simulink model "Quadrotor_Model"  (R2025b)
settings: Solver=ode45  StartTime=0.0  StopTime=15000  RelTol=1e-3  EnableMultiTasking=on
values from neighbouring files (symbols this model uses):
  b = 0.07    [project_launch.m]
  g = 9.81    [project_launch.m]
  Ixx = (2/5) * m_drone * r_body^2 + 2 * L^2 * m_motor    (= 0.0145321875)    [project_launch.m]
  Iyy = Ixx    (= 0.0145321875)    [project_launch.m]
  Izz = (2/5) * m_drone * r_body^2 + 4 * L^2 * m_motor    (= 0.0270321875)    [project_launch.m]
  Jr = 0.01 * m_motor * r_prop^2    (= 1.6129e-05)    [project_launch.m]
  k = 0.09    [project_launch.m]
  K_d_phi = 8    [project_launch.m]
  K_d_psi = 4    [project_launch.m]
  K_d_theta = 8    [project_launch.m]
  K_dx = 1.2    [project_launch.m]
  K_dy = 1.2    [project_launch.m]
  K_dz = 1.8    [project_launch.m]
  K_p_phi = 25    [project_launch.m]
  K_p_psi = 9    [project_launch.m]
  K_p_theta = 25    [project_launch.m]
  K_px = 0.6    [project_launch.m]
  K_py = 0.6    [project_launch.m]
  K_pz = 1.2    [project_launch.m]
  L = 0.25    [project_launch.m]
  m = 1.7006    [project_launch.m]
  tau_v = 0.1    [project_launch.m]
settings Model: Creator=boyan  LastModifiedBy=89286
settings SolverCC: MaxConsecutiveMinStep=2  AlgebraicLoopSolver=TrustRegion
settings DataIOCC: LimitDataPoints=on  SaveFormat=Array  ReturnWorkspaceOutputs=off
settings OptimizationCC: LifeSpan=inf
settings DebuggingCC: SolverPrmCheckMsg=warning  UnconnectedInputMsg=warning  UnconnectedOutputMsg=warning  UnconnectedLineMsg=warning  SFUnexpectedBacktrackingDiag=warning  SFNoUnconditionalDefaultTransitionDiag=warning  SFExecutionAtInitializationDiag=none  ArithmeticOperatorsInVariantConditions=warning
settings HardwareCC: ProdBitPerPointer=32.0  ProdBitPerSizeT=32.0  ProdBitPerPtrDiffT=32.0  ProdLargestAtomicFloat=None  ProdIntDivRoundTo=Undefined  ProdEndianess=Unspecified  ProdWordSize=32.0  ProdHWDeviceType=32-bit Generic
settings ModelReferenceCC: EnableRefExpFcnMdlSchedulingChecks=on  PropagateSignalLabelsOutOfModel=off
settings SFSimCC: SimUseLocalCustomCode=off  CustomCodeUndefinedFunction=UseInterfaceOnly
settings RTWCC: RTWUseLocalCustomCode=off  GPUComputeCapability=3.5  DLArmComputeVersion=19.05
settings CodeAppCC: StateflowObjectComments=on
settings GRTTargetCC: TargetLangStandard=C89/C90 (ANSI)
settings ConfigComp: CovMetricSettings=dw  CovSaveCumulativeToWorkspaceVar=on  CovSaveSingleToWorkspaceVar=on  CovExternalEMLEnable=off  CovSFcnEnable=off

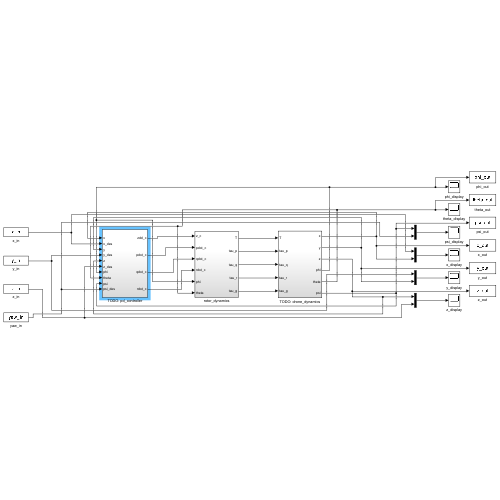
[thumbnail: Simulink's stored preview of the top-level diagram]
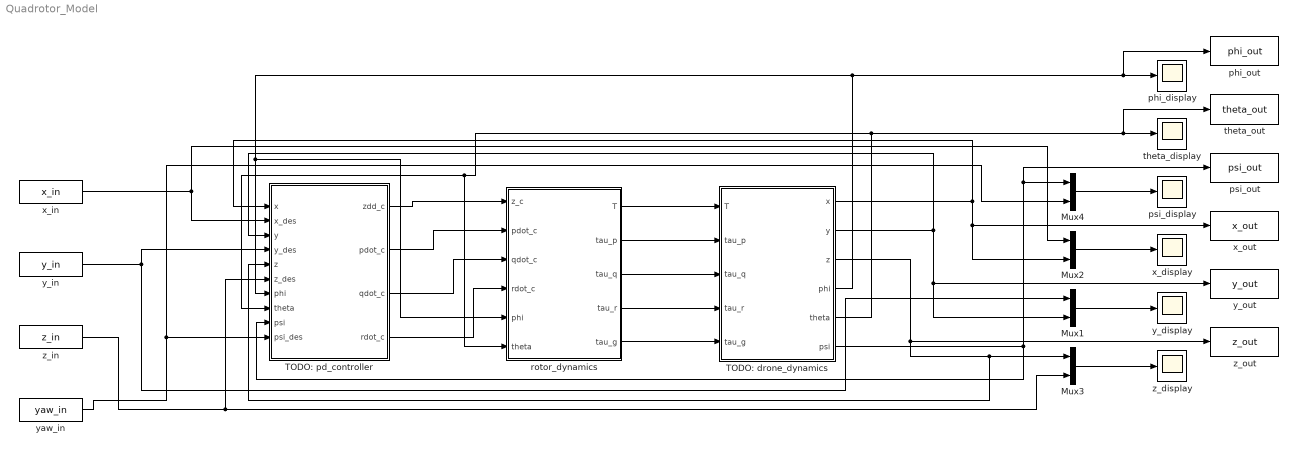
== system Quadrotor_Model ==
  Mux{1..4} (4 alike) : Mux  Inputs=2
  TODO: drone_dynamics : Subsystem
  TODO: pd_controller : Subsystem
  phi_display : Scope
      settings: ActiveDisplayYMinimum=-48.30659  ActiveDisplayYMaximum=31.01137
  phi_out : ToWorkspace  VariableName=phi_out  SaveFormat=Timeseries  SampleTime=-1
  psi_display : Scope
      settings: ActiveDisplayYMinimum=-104019.46579  ActiveDisplayYMaximum=26220.25866  DataLoggingVariableName=ScopeData2
  psi_out : ToWorkspace  VariableName=psi_out  SaveFormat=Timeseries  SampleTime=-1
  rotor_dynamics : Subsystem
  theta_display : Scope
      settings: ActiveDisplayYMinimum=-1.26378  ActiveDisplayYMaximum=0.84614  DataLoggingVariableName=ScopeData3
  theta_out : ToWorkspace  VariableName=theta_out  SaveFormat=Timeseries  SampleTime=-1
  x_display : Scope
      settings: ActiveDisplayYMinimum=-0.02581  ActiveDisplayYMaximum=0.17972  DataLoggingVariableName=ScopeData4
  x_in : FromWorkspace  VariableName=x_in
  x_out : ToWorkspace  VariableName=x_out  SaveFormat=Timeseries  SampleTime=-1
  y_display : Scope
      settings: ActiveDisplayYMinimum=98.09651  ActiveDisplayYMaximum=101.74643  DataLoggingVariableName=ScopeData5
  y_in : FromWorkspace  VariableName=y_in
  y_out : ToWorkspace  VariableName=y_out  SaveFormat=Timeseries  SampleTime=-1
  yaw_in : FromWorkspace  VariableName=yaw_in
  z_display : Scope
      settings: ActiveDisplayYMinimum=-47.57242  ActiveDisplayYMaximum=5.28582
  z_in : FromWorkspace  VariableName=z_in
  z_out : ToWorkspace  VariableName=z_out  SaveFormat=Timeseries  SampleTime=-1
  wires:
  rotor_dynamics/1(T) -> TODO: drone_dynamics/1(T)
  rotor_dynamics/2(tau_p) -> TODO: drone_dynamics/2(tau_p)
  TODO: pd_controller/1(zdd_c) -> rotor_dynamics/1(z_c)
  TODO: pd_controller/2(pdot_c) -> rotor_dynamics/2(pdot_c)
  z_in/1 -> TODO: pd_controller/6(z_des), Mux3/2
  Mux1/1 -> y_display/1
  Mux2/1 -> x_display/1
  Mux4/1 -> psi_display/1
  Mux3/1 -> z_display/1
  TODO: drone_dynamics/6(psi) -> TODO: pd_controller/9(psi), psi_out/1, Mux4/1
  y_in/1 -> TODO: pd_controller/4(y_des), Mux1/1
  x_in/1 -> TODO: pd_controller/2(x_des), Mux2/1
  TODO: drone_dynamics/3(z) -> z_out/1, TODO: pd_controller/5(z), Mux3/1
  TODO: drone_dynamics/5(theta) -> theta_out/1, theta_display/1, rotor_dynamics/6(theta), TODO: pd_controller/8(theta)
  TODO: drone_dynamics/2(y) -> TODO: pd_controller/3(y), Mux1/2, y_out/1
  TODO: drone_dynamics/4(phi) -> phi_out/1, phi_display/1, rotor_dynamics/5(phi), TODO: pd_controller/7(phi)
  TODO: drone_dynamics/1(x) -> TODO: pd_controller/1(x), Mux2/2, x_out/1
  rotor_dynamics/5(tau_g) -> TODO: drone_dynamics/5(tau_g)
  rotor_dynamics/3(tau_q) -> TODO: drone_dynamics/3(tau_q)
  rotor_dynamics/4(tau_r) -> TODO: drone_dynamics/4(tau_r)
  yaw_in/1 -> TODO: pd_controller/10(psi_des), Mux4/2
  TODO: pd_controller/4(rdot_c) -> rotor_dynamics/4(rdot_c)
  TODO: pd_controller/3(qdot_c) -> rotor_dynamics/3(qdot_c)

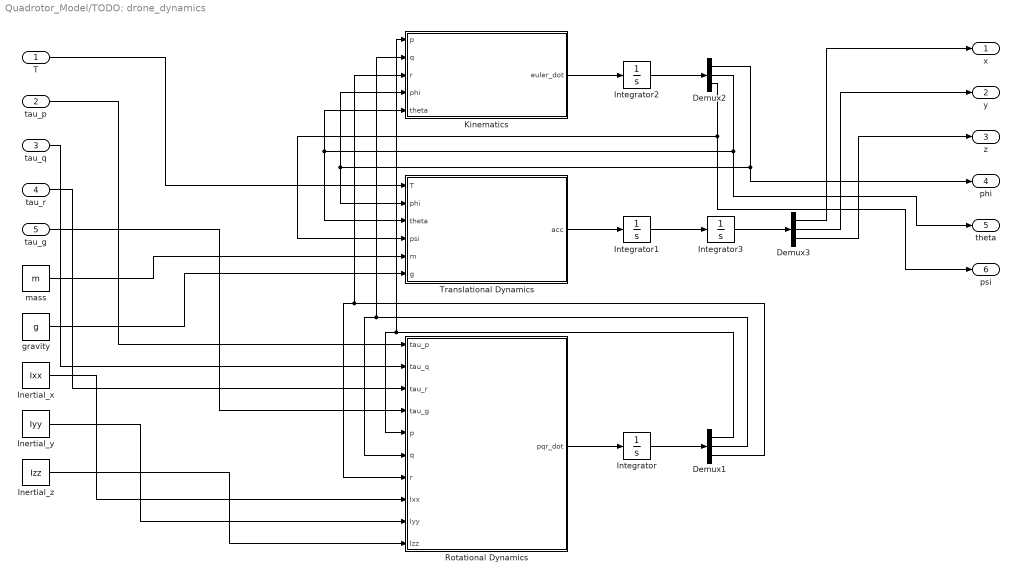
== system Quadrotor_Model/TODO: drone_dynamics ==
  T : Inport
  tau_p : Inport  Port=2
  tau_q : Inport  Port=3
  tau_r : Inport  Port=4
  tau_g : Inport  Port=5
  Demux1 : Demux  Outputs=3
  Demux2 : Demux  Outputs=3
  Demux3 : Demux  Outputs=3
  Inertial_x : Constant  Value=Ixx
  Inertial_y : Constant  Value=Iyy
  Inertial_z : Constant  Value=Izz
  Integrator{,1..3} (4 alike) : Integrator
  Kinematics : MATLAB Function  TreatAsAtomicUnit=on
  Rotational Dynamics : MATLAB Function  TreatAsAtomicUnit=on
  Translational Dynamics : MATLAB Function  TreatAsAtomicUnit=on
  gravity : Constant  Value=g
  mass : Constant  Value=m
  x : Outport
  y : Outport  Port=2
  z : Outport  Port=3
  phi : Outport  Port=4
  theta : Outport  Port=5
  psi : Outport  Port=6
  wires:
  mass/1 -> Translational Dynamics/5(m)
  gravity/1 -> Translational Dynamics/6(g)
  Inertial_x/1 -> Rotational Dynamics/8(Ixx)
  Inertial_y/1 -> Rotational Dynamics/9(Iyy)
  Inertial_z/1 -> Rotational Dynamics/10(Izz)
  T/1 -> Translational Dynamics/1(T)
  tau_p/1 -> Rotational Dynamics/1(tau_p)
  tau_q/1 -> Rotational Dynamics/2(tau_q)
  tau_r/1 -> Rotational Dynamics/3(tau_r)
  tau_g/1 -> Rotational Dynamics/4(tau_g)
  Translational Dynamics/1(acc) -> Integrator1/1
  Rotational Dynamics/1(pqr_dot) -> Integrator/1
  Integrator/1 -> Demux1/1
  Integrator1/1 -> Integrator3/1
  Demux1/1 -> Kinematics/1(p), Rotational Dynamics/5(p)
  Demux1/2 -> Kinematics/2(q), Rotational Dynamics/6(q)
  Demux1/3 -> Kinematics/3(r), Rotational Dynamics/7(r)
  Kinematics/1(euler_dot) -> Integrator2/1
  Integrator2/1 -> Demux2/1
  Integrator3/1 -> Demux3/1
  Demux3/1 -> x/1
  Demux3/2 -> y/1
  Demux3/3 -> z/1
  Demux2/1 -> phi/1, Kinematics/4(phi), Translational Dynamics/2(phi)
  Demux2/2 -> theta/1, Translational Dynamics/3(theta), Kinematics/5(theta)
  Demux2/3 -> Translational Dynamics/4(psi), psi/1

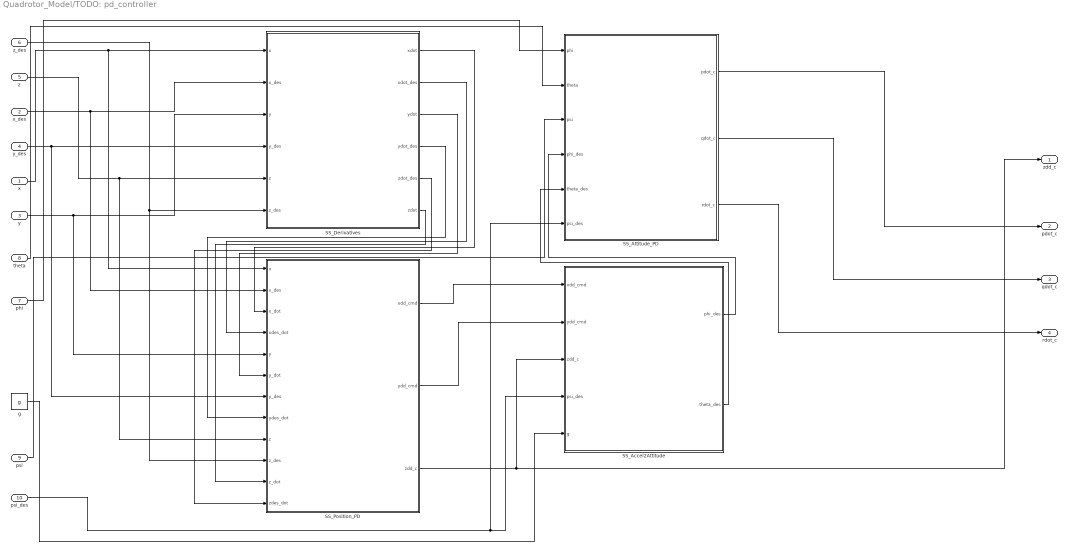
== system Quadrotor_Model/TODO: pd_controller ==
  x : Inport
  x_des : Inport  Port=2
  y : Inport  Port=3
  y_des : Inport  Port=4
  z : Inport  Port=5
  z_des : Inport  Port=6
  phi : Inport  Port=7
  theta : Inport  Port=8
  psi : Inport  Port=9
  psi_des : Inport  Port=10
  SS_Accel2Attitude : Subsystem
  SS_Attitude_PD : Subsystem
  SS_Derivatives : Subsystem
  SS_Position_PD : Subsystem
  g : Constant  Value=g
  zdd_c : Outport
  pdot_c : Outport  Port=2
  qdot_c : Outport  Port=3
  rdot_c : Outport  Port=4
  wires:
  x/1 -> SS_Position_PD/1(x), SS_Derivatives/1(x)
  x_des/1 -> SS_Position_PD/2(x_des), SS_Derivatives/2(x_des)
  z_des/1 -> SS_Position_PD/10(z_des), SS_Derivatives/6(z_des)
  z/1 -> SS_Derivatives/5(z), SS_Position_PD/9(z)
  y_des/1 -> SS_Position_PD/7(y_des), SS_Derivatives/4(y_des)
  y/1 -> SS_Position_PD/5(y), SS_Derivatives/3(y)
  SS_Position_PD/3(zdd_c) -> SS_Accel2Attitude/3(zdd_c), zdd_c/1
  SS_Position_PD/1(xdd_cmd) -> SS_Accel2Attitude/1(xdd_cmd)
  SS_Position_PD/2(ydd_cmd) -> SS_Accel2Attitude/2(ydd_cmd)
  g/1 -> SS_Accel2Attitude/5(g)
  psi_des/1 -> SS_Attitude_PD/6(psi_des), SS_Accel2Attitude/4(psi_des)
  SS_Derivatives/1(xdot) -> SS_Position_PD/3(x_dot)
  SS_Derivatives/2(xdot_des) -> SS_Position_PD/4(xdes_dot)
  SS_Derivatives/3(ydot) -> SS_Position_PD/6(y_dot)
  SS_Derivatives/4(ydot_des) -> SS_Position_PD/8(ydes_dot)
  SS_Derivatives/5(zdot_des) -> SS_Position_PD/12(zdes_dot)
  SS_Derivatives/6(zdot) -> SS_Position_PD/11(z_dot)
  SS_Attitude_PD/1(pdot_c) -> pdot_c/1
  SS_Attitude_PD/2(qdot_c) -> qdot_c/1
  SS_Attitude_PD/3(rdot_c) -> rdot_c/1
  SS_Accel2Attitude/1(phi_des) -> SS_Attitude_PD/4(phi_des)
  SS_Accel2Attitude/2(theta_des) -> SS_Attitude_PD/5(theta_des)
  psi/1 -> SS_Attitude_PD/3(psi)
  phi/1 -> SS_Attitude_PD/1(phi)
  theta/1 -> SS_Attitude_PD/2(theta)

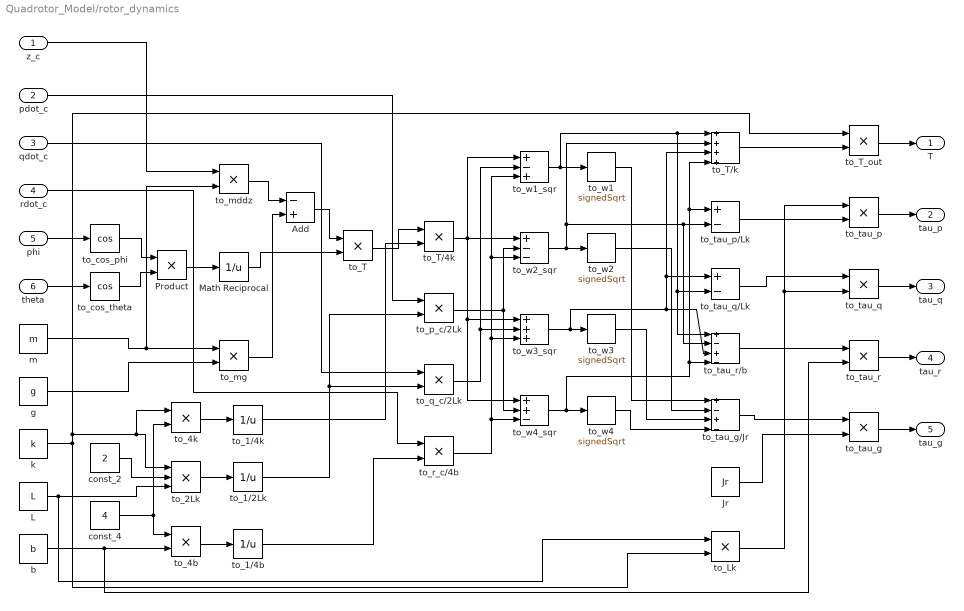
== system Quadrotor_Model/rotor_dynamics ==
  z_c : Inport
  pdot_c : Inport  Port=2
  qdot_c : Inport  Port=3
  rdot_c : Inport  Port=4
  phi : Inport  Port=5
  theta : Inport  Port=6
  Add : Sum  Inputs=-+
  Jr : Constant  Value=Jr
  L : Constant  Value=L
  Math Reciprocal : Math  Operator=reciprocal  SignedPower=on
  Product : Product
  b : Constant  Value=b
  const_2 : Constant  Value=2
  const_4 : Constant  Value=4
  g : Constant  Value=g
  k : Constant  Value=k
  m : Constant  Value=m
  to_1/2Lk : Math  Operator=reciprocal  SignedPower=on
  to_1/4b : Math  Operator=reciprocal  SignedPower=on
  to_1/4k : Math  Operator=reciprocal  SignedPower=on
  to_2Lk : Product  Inputs=3
  to_4b : Product
  to_4k : Product
  to_Lk : Product
  to_T : Product
  to_T/4k : Product
  to_T/k : Sum  Inputs=++++
  to_T_out : Product
  to_cos_phi : Trigonometry  Operator=cos
  to_cos_theta : Trigonometry  Operator=cos
  to_mddz : Product
  to_mg : Product
  to_p_c/2Lk : Product
  to_q_c/2Lk : Product
  to_r_c/4b : Product
  to_tau_g : Product
  to_tau_g/Jr : Sum  Inputs=+-+-
  to_tau_p : Product
  to_tau_p/Lk : Sum  Inputs=+-
  to_tau_q : Product
  to_tau_q/Lk : Sum  Inputs=+-
  to_tau_r : Product
  to_tau_r/b : Sum  Inputs=+-+-
  to_w{1..4} (4 alike) : Sqrt  Operator=signedSqrt
  to_w1_sqr : Sum  Inputs=+-+
  to_w2_sqr : Sum  Inputs=+--
  to_w3_sqr : Sum  Inputs=+++
  to_w4_sqr : Sum  Inputs=++-
  T : Outport
  tau_p : Outport  Port=2
  tau_q : Outport  Port=3
  tau_r : Outport  Port=4
  tau_g : Outport  Port=5
  wires:
  phi/1 -> to_cos_phi/1
  theta/1 -> to_cos_theta/1
  to_cos_phi/1 -> Product/1
  to_cos_theta/1 -> Product/2
  Product/1 -> Math Reciprocal/1
  m/1 -> to_mddz/2, to_mg/1
  g/1 -> to_mg/2
  to_mg/1 -> Add/2
  Math Reciprocal/1 -> to_T/2
  Add/1 -> to_T/1
  k/1 -> to_2Lk/1, to_4k/1, to_T_out/1, to_Lk/2
  const_4/1 -> to_4b/1, to_4k/2
  const_2/1 -> to_2Lk/2
  L/1 -> to_2Lk/3, to_Lk/1
  b/1 -> to_tau_r/2, to_4b/2
  to_4k/1 -> to_1/4k/1
  to_2Lk/1 -> to_1/2Lk/1
  to_4b/1 -> to_1/4b/1
  to_T/1 -> to_T/4k/1
  to_1/4k/1 -> to_T/4k/2
  pdot_c/1 -> to_p_c/2Lk/1
  to_1/2Lk/1 -> to_q_c/2Lk/2, to_p_c/2Lk/2
  qdot_c/1 -> to_q_c/2Lk/1
  to_1/4b/1 -> to_r_c/4b/2
  rdot_c/1 -> to_r_c/4b/1
  to_T/4k/1 -> to_w2_sqr/1, to_w3_sqr/1, to_w4_sqr/1, to_w1_sqr/1
  to_q_c/2Lk/1 -> to_w3_sqr/2, to_w1_sqr/2
  to_r_c/4b/1 -> to_w4_sqr/3, to_w3_sqr/3, to_w2_sqr/3, to_w1_sqr/3
  to_p_c/2Lk/1 -> to_w2_sqr/2, to_w4_sqr/2
  to_w1_sqr/1 -> to_w1/1, to_tau_r/b/1, to_tau_q/Lk/2, to_T/k/1
  to_w2_sqr/1 -> to_w2/1, to_tau_r/b/2, to_tau_p/Lk/2, to_T/k/2
  to_w3_sqr/1 -> to_w3/1, to_tau_q/Lk/1, to_T/k/3, to_tau_r/b/3
  to_w4_sqr/1 -> to_w4/1, to_tau_p/Lk/1, to_T/k/4, to_tau_r/b/4
  to_w2/1 -> to_tau_g/Jr/2
  to_w1/1 -> to_tau_g/Jr/1
  to_w3/1 -> to_tau_g/Jr/3
  to_w4/1 -> to_tau_g/Jr/4
  to_T_out/1 -> T/1
  to_T/k/1 -> to_T_out/2
  to_tau_p/1 -> tau_p/1
  to_tau_p/Lk/1 -> to_tau_p/2
  to_tau_q/1 -> tau_q/1
  to_tau_r/1 -> tau_r/1
  to_tau_r/b/1 -> to_tau_r/1
  to_tau_q/Lk/1 -> to_tau_q/1
  to_tau_g/1 -> tau_g/1
  to_Lk/1 -> to_tau_p/1, to_tau_q/2
  Jr/1 -> to_tau_g/2
  z_c/1 -> to_mddz/1
  to_mddz/1 -> Add/1
  to_tau_g/Jr/1 -> to_tau_g/1

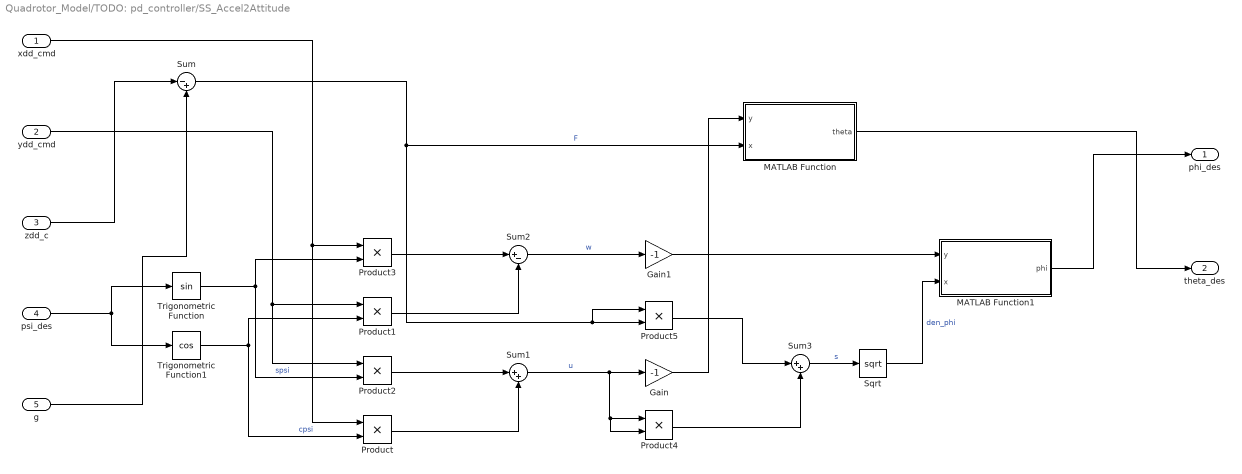
== system Quadrotor_Model/TODO: pd_controller/SS_Accel2Attitude ==
  xdd_cmd : Inport
  ydd_cmd : Inport  Port=2
  zdd_c : Inport  Port=3
  psi_des : Inport  Port=4
  g : Inport  Port=5
  Gain : Gain  Gain=-1
  Gain1 : Gain  Gain=-1
  MATLAB Function : MATLAB Function  TreatAsAtomicUnit=on
  MATLAB Function1 : MATLAB Function  TreatAsAtomicUnit=on
  Product{,1..5} (6 alike) : Product
  Sqrt : Sqrt
  Sum : Sum  Inputs=|-+
  Sum1 : Sum  Inputs=|++
  Sum2 : Sum  Inputs=|+-
  Sum3 : Sum  Inputs=|++
  Trigonometric Function : Trigonometry
  Trigonometric Function1 : Trigonometry  Operator=cos
  phi_des : Outport
  theta_des : Outport  Port=2
  wires:
  psi_des/1 -> Trigonometric Function1/1, Trigonometric Function/1
  Trigonometric Function/1 -> Product2/2, Product3/2  "spsi"
  Trigonometric Function1/1 -> Product1/2, Product/2  "cpsi"
  g/1 -> Sum/2
  zdd_c/1 -> Sum/1
  Sum/1 -> Product5/1, Product5/2, MATLAB Function/2(x)  "F"
  xdd_cmd/1 -> Product3/1, Product/1
  ydd_cmd/1 -> Product1/1, Product2/1
  Product2/1 -> Sum1/1
  Product/1 -> Sum1/2
  Sum1/1 -> Product4/2, Product4/1, Gain/1  "u"
  Product1/1 -> Sum2/2
  Product3/1 -> Sum2/1
  Sum2/1 -> Gain1/1  "w"
  Gain/1 -> MATLAB Function/1(y)
  Gain1/1 -> MATLAB Function1/1(y)
  MATLAB Function1/1(phi) -> phi_des/1
  MATLAB Function/1(theta) -> theta_des/1
  Product5/1 -> Sum3/1
  Product4/1 -> Sum3/2
  Sum3/1 -> Sqrt/1  "s"
  Sqrt/1 -> MATLAB Function1/2(x)  "den_phi"

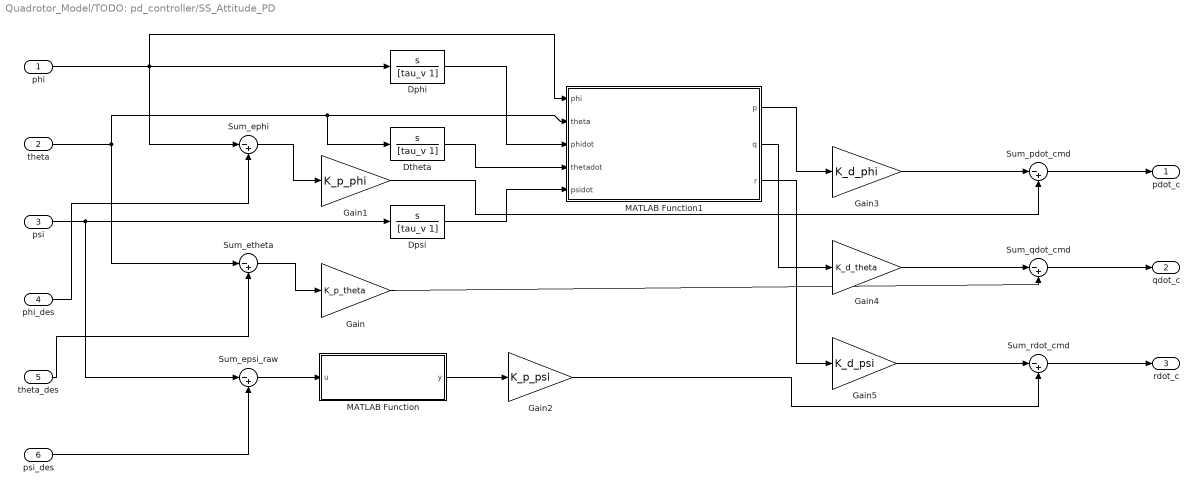
== system Quadrotor_Model/TODO: pd_controller/SS_Attitude_PD ==
  phi : Inport
  theta : Inport  Port=2
  psi : Inport  Port=3
  phi_des : Inport  Port=4
  theta_des : Inport  Port=5
  psi_des : Inport  Port=6
  Dphi : TransferFcn  Numerator=[1 0]  Denominator=[tau_v 1]
  Dpsi : TransferFcn  Numerator=[1 0]  Denominator=[tau_v 1]
  Dtheta : TransferFcn  Numerator=[1 0]  Denominator=[tau_v 1]
  Gain : Gain  Gain=K_p_theta
  Gain1 : Gain  Gain=K_p_phi
  Gain2 : Gain  Gain=K_p_psi
  Gain3 : Gain  Gain=K_d_phi
  Gain4 : Gain  Gain=K_d_theta
  Gain5 : Gain  Gain=K_d_psi
  MATLAB Function : MATLAB Function  TreatAsAtomicUnit=on
  MATLAB Function1 : MATLAB Function  TreatAsAtomicUnit=on
  Sum_ephi : Sum  Inputs=|-+
  Sum_epsi_raw : Sum  Inputs=|-+
  Sum_etheta : Sum  Inputs=|-+
  Sum_pdot_cmd : Sum  Inputs=|-+
  Sum_qdot_cmd : Sum  Inputs=|-+
  Sum_rdot_cmd : Sum  Inputs=|-+
  pdot_c : Outport
  qdot_c : Outport  Port=2
  rdot_c : Outport  Port=3
  wires:
  phi/1 -> Sum_ephi/1, MATLAB Function1/1(phi), Dphi/1
  phi_des/1 -> Sum_ephi/2
  theta_des/1 -> Sum_etheta/2
  theta/1 -> Sum_etheta/1, Dtheta/1, MATLAB Function1/2(theta)
  psi/1 -> Sum_epsi_raw/1, Dpsi/1
  psi_des/1 -> Sum_epsi_raw/2
  Sum_epsi_raw/1 -> MATLAB Function/1(u)
  MATLAB Function/1(y) -> Gain2/1
  Dphi/1 -> MATLAB Function1/3(phidot)
  Dtheta/1 -> MATLAB Function1/4(thetadot)
  Dpsi/1 -> MATLAB Function1/5(psidot)
  Sum_etheta/1 -> Gain/1
  Sum_ephi/1 -> Gain1/1
  MATLAB Function1/1(p) -> Gain3/1
  MATLAB Function1/2(q) -> Gain4/1
  MATLAB Function1/3(r) -> Gain5/1
  Gain3/1 -> Sum_pdot_cmd/1
  Gain4/1 -> Sum_qdot_cmd/1
  Gain5/1 -> Sum_rdot_cmd/1
  Gain1/1 -> Sum_pdot_cmd/2
  Gain/1 -> Sum_qdot_cmd/2
  Gain2/1 -> Sum_rdot_cmd/2
  Sum_rdot_cmd/1 -> rdot_c/1
  Sum_qdot_cmd/1 -> qdot_c/1
  Sum_pdot_cmd/1 -> pdot_c/1

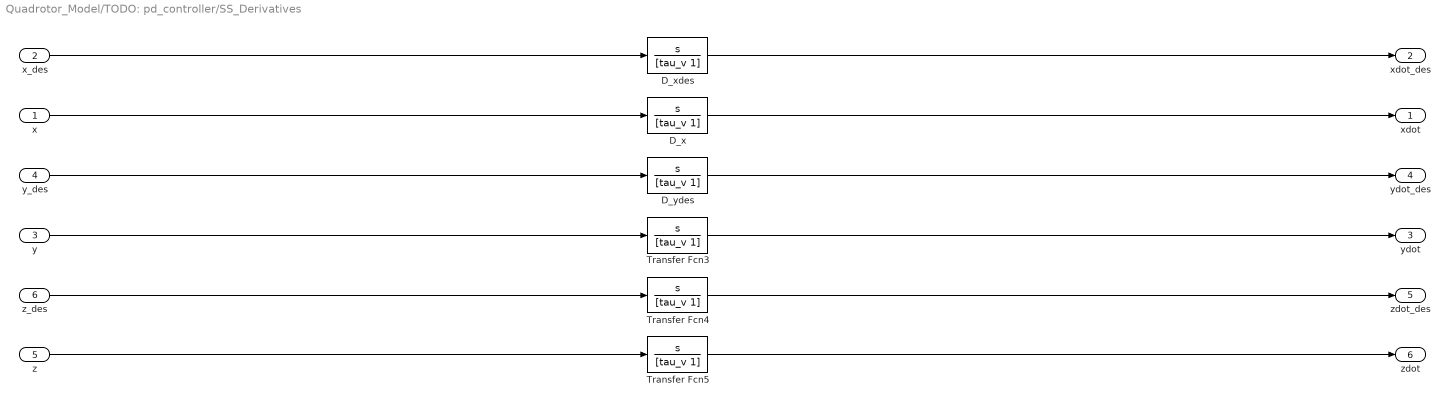
== system Quadrotor_Model/TODO: pd_controller/SS_Derivatives ==
  x : Inport
  x_des : Inport  Port=2
  y : Inport  Port=3
  y_des : Inport  Port=4
  z : Inport  Port=5
  z_des : Inport  Port=6
  D_x : TransferFcn  Numerator=[1 0]  Denominator=[tau_v 1]
  D_xdes : TransferFcn  Numerator=[1 0]  Denominator=[tau_v 1]
  D_ydes : TransferFcn  Numerator=[1 0]  Denominator=[tau_v 1]
  Transfer Fcn3 : TransferFcn  Numerator=[1 0]  Denominator=[tau_v 1]
  Transfer Fcn4 : TransferFcn  Numerator=[1 0]  Denominator=[tau_v 1]
  Transfer Fcn5 : TransferFcn  Numerator=[1 0]  Denominator=[tau_v 1]
  xdot : Outport
  xdot_des : Outport  Port=2
  ydot : Outport  Port=3
  ydot_des : Outport  Port=4
  zdot_des : Outport  Port=5
  zdot : Outport  Port=6
  wires:
  x/1 -> D_x/1
  D_x/1 -> xdot/1
  x_des/1 -> D_xdes/1
  D_xdes/1 -> xdot_des/1
  y_des/1 -> D_ydes/1
  D_ydes/1 -> ydot_des/1
  y/1 -> Transfer Fcn3/1
  Transfer Fcn3/1 -> ydot/1
  z_des/1 -> Transfer Fcn4/1
  Transfer Fcn4/1 -> zdot_des/1
  z/1 -> Transfer Fcn5/1
  Transfer Fcn5/1 -> zdot/1

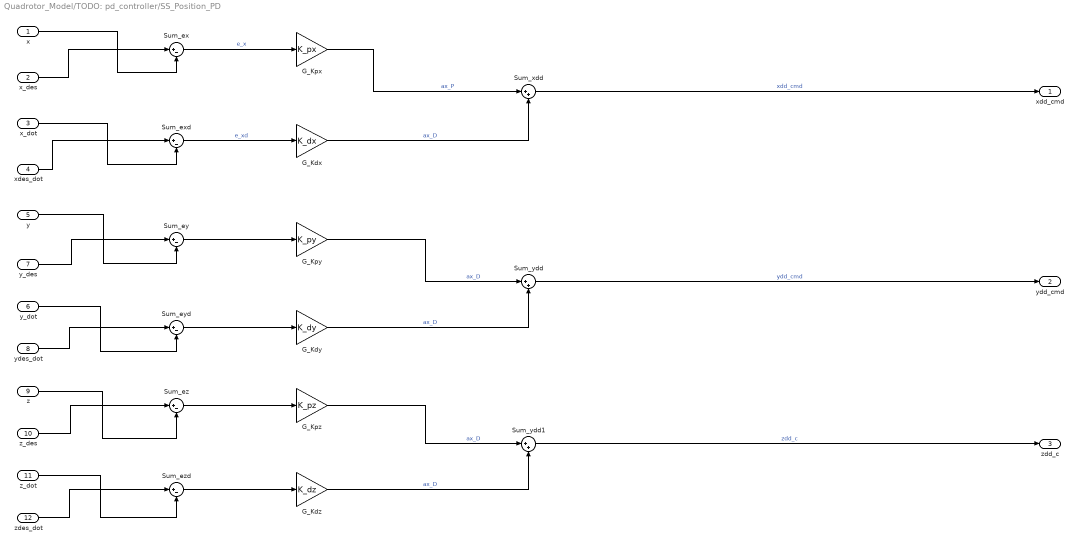
== system Quadrotor_Model/TODO: pd_controller/SS_Position_PD ==
  x : Inport
  x_des : Inport  Port=2
  x_dot : Inport  Port=3
  xdes_dot : Inport  Port=4
  y : Inport  Port=5
  y_dot : Inport  Port=6
  y_des : Inport  Port=7
  ydes_dot : Inport  Port=8
  z : Inport  Port=9
  z_des : Inport  Port=10
  z_dot : Inport  Port=11
  zdes_dot : Inport  Port=12
  G_Kdx : Gain  Gain=K_dx
  G_Kdy : Gain  Gain=K_dy
  G_Kdz : Gain  Gain=K_dz
  G_Kpx : Gain  Gain=K_px
  G_Kpy : Gain  Gain=K_py
  G_Kpz : Gain  Gain=K_pz
  Sum_ex : Sum  Inputs=|+-
  Sum_exd : Sum  Inputs=|+-
  Sum_ey : Sum  Inputs=|+-
  Sum_eyd : Sum  Inputs=|+-
  Sum_ez : Sum  Inputs=|+-
  Sum_ezd : Sum  Inputs=|+-
  Sum_xdd : Sum  Inputs=|++
  Sum_ydd : Sum  Inputs=|++
  Sum_ydd1 : Sum  Inputs=|++
  xdd_cmd : Outport
  ydd_cmd : Outport  Port=2
  zdd_c : Outport  Port=3
  wires:
  x_des/1 -> Sum_ex/1
  x/1 -> Sum_ex/2
  Sum_ex/1 -> G_Kpx/1  "e_x"
  x_dot/1 -> Sum_exd/2
  xdes_dot/1 -> Sum_exd/1
  Sum_exd/1 -> G_Kdx/1  "e_xd"
  G_Kdx/1 -> Sum_xdd/2  "ax_D"
  G_Kpx/1 -> Sum_xdd/1  "ax_P"
  Sum_xdd/1 -> xdd_cmd/1  "xdd_cmd"
  y/1 -> Sum_ey/2
  y_des/1 -> Sum_ey/1
  y_dot/1 -> Sum_eyd/2
  ydes_dot/1 -> Sum_eyd/1
  Sum_ey/1 -> G_Kpy/1
  Sum_eyd/1 -> G_Kdy/1
  G_Kpy/1 -> Sum_ydd/1  "ax_D"
  G_Kdy/1 -> Sum_ydd/2  "ax_D"
  Sum_ydd/1 -> ydd_cmd/1  "ydd_cmd"
  z/1 -> Sum_ez/2
  z_des/1 -> Sum_ez/1
  z_dot/1 -> Sum_ezd/2
  zdes_dot/1 -> Sum_ezd/1
  Sum_ez/1 -> G_Kpz/1
  Sum_ezd/1 -> G_Kdz/1
  G_Kpz/1 -> Sum_ydd1/1  "ax_D"
  G_Kdz/1 -> Sum_ydd1/2  "ax_D"
  Sum_ydd1/1 -> zdd_c/1  "zdd_c"

== matlab function Quadrotor_Model/TODO: drone_dynamics/Rotational Dynamics ==
  data: tau_p input; pqr_dot output; tau_q input; tau_r input; tau_g input; p input; q input; r input; Ixx input; Iyy input; Izz input
function pqr_dot = Rotational_Dyn(tau_p, tau_q, tau_r, tau_g, p, q, r, Ixx, Iyy, Izz)

pqr_dot = zeros(3,1);

pqr_dot(1) = (1/Ixx) * (tau_p + q * tau_g + (Iyy - Izz) * q * r);

pqr_dot(2) = (1/Iyy) * (tau_q - p * tau_g + (Izz - Ixx) * p * r);

pqr_dot(3) = (1/Izz) * (tau_r + (Ixx - Iyy) * p * q);

end

== matlab function Quadrotor_Model/TODO: drone_dynamics/Translational Dynamics ==
  data: acc output; T input; phi input; theta input; psi input; m input; g input
function acc = Translational_Dyn(T, phi, theta, psi, m, g)
% Translational acceleration in NED frame (positive Down)
% a = g*e3 - (T/m) * R(:,3), with R = Rz(psi)Ry(theta)Rx(phi)

acc = zeros(3,1);

acc(1) = -T/m * (cos(psi)*sin(theta)*cos(phi) + sin(psi)*sin(phi));
acc(2) = -T/m * (sin(psi)*sin(theta)*cos(phi) - cos(psi)*sin(phi));
acc(3) =  g   - T/m * (cos(theta)*cos(phi));

end

== matlab function Quadrotor_Model/TODO: drone_dynamics/Kinematics ==
  data: p input; euler_dot output; q input; r input; phi input; theta input
function euler_dot = Kinematics(p, q, r, phi, theta)

euler_dot = attitude_compdyn([phi, theta], [p; q; r]);

end

== matlab function Quadrotor_Model/TODO: pd_controller/SS_Accel2Attitude/MATLAB Function ==
  data: y input; theta output; x input
function theta = atan2_theta(y,x)
theta = atan2(y,x);
end

== matlab function Quadrotor_Model/TODO: pd_controller/SS_Accel2Attitude/MATLAB Function1 ==
  data: y input; phi output; x input
function phi = atan2_phi(y,x)
phi = atan2(y,x);
end

== matlab function Quadrotor_Model/TODO: pd_controller/SS_Attitude_PD/MATLAB Function ==
  data: u input; y output
function y = wrapToPi(u)
% Wrap angle to (-pi, pi]
y = atan2(sin(u), cos(u));
end

== matlab function Quadrotor_Model/TODO: pd_controller/SS_Attitude_PD/MATLAB Function1 ==
  data: phi input; p output; theta input; phidot input; thetadot input; psidot input; q output; r output
function [p,q,r] = EulerDot2PQR(phi, theta, phidot, thetadot, psidot)
% ZYX Euler rates -> body rates (p,q,r)
p = phidot - psidot*sin(theta);
q = thetadot*cos(phi) + psidot*sin(phi)*cos(theta);
r = -thetadot*sin(phi) + psidot*cos(phi)*cos(theta);
end
